simulink model "gm_mult_1"  (R2023a)
settings: Solver=FixedStepDiscrete  StartTime=0.0  StopTime=10.0  RelTol=1e-3
undefined symbols (not defined in the file or in its folder): dt
libraries: simulink x1
settings Model: Creator=szymadej  LastModifiedBy=szymadej
settings OptimizationCC: BlockReduction=off  ConditionallyExecuteInputs=off  DefaultParameterBehavior=Inlined  InheritOutputTypeSmallerThanSingle=on
settings DebuggingCC: AlgebraicLoopMsg=error  InheritedTsInSrcMsg=none  SingleTaskRateTransMsg=error  UnconnectedInputMsg=warning  UnconnectedOutputMsg=warning  UnconnectedLineMsg=warning
settings HardwareCC: ProdBitPerPointer=32  ProdBitPerSizeT=32  ProdBitPerPtrDiffT=32  ProdLargestAtomicFloat=None  ProdIntDivRoundTo=Undefined  ProdEndianess=Unspecified  ProdWordSize=32  ProdHWDeviceType=ASIC/FPGA->ASIC/FPGA  TargetBitPerLong=64  TargetBitPerPointer=64  TargetBitPerSizeT=64  TargetBitPerPtrDiffT=64  TargetLongLongMode=on  TargetIntDivRoundTo=Zero  TargetEndianess=LittleEndian  TargetWordSize=64  TargetHWDeviceType=Custom Processor->MATLAB Host Computer  ProdEqTarget=off

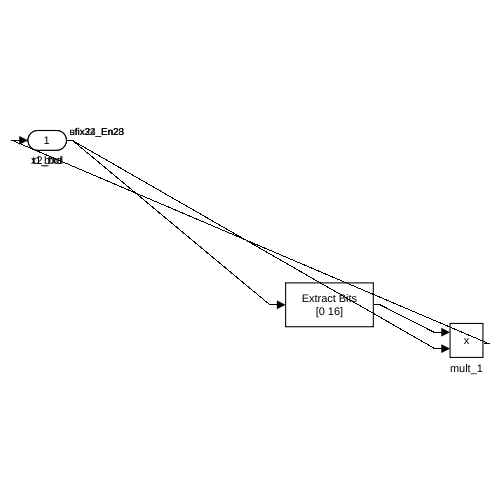
[thumbnail: Simulink's stored preview of the top-level diagram]
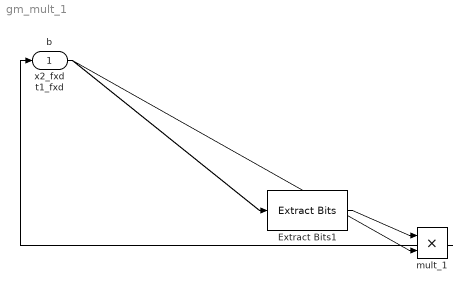
== system gm_mult_1 ==
  x2_fxd : Inport  OutDataTypeStr=fixdt(0, 24, 23)  PortDimensions=1  SampleTime=0.2
  b : Inport  Port=2  OutDataTypeStr=fixdt(1, 32, 28)  PortDimensions=1  SampleTime=0.2
  Extract Bits1 : simulink/Logic and Bit Operations/Extract Bits  bitsToExtract=Range of bits  numBits=17  bitIdxRange=[0 dt.x2_fxd.w-1]  outScalingMode=Preserve fixed-point scaling
  mult_1 : Product  OutDataTypeStr=fixdt(dt.t1_fxd.s,dt.t1_fxd.w,dt.t1_fxd.f)
  t1_fxd : Outport  SampleTime=0.2
  wires:
  x2_fxd/1 -> Extract Bits1/1
  b/1 -> mult_1/2
  Extract Bits1/1 -> mult_1/1
  mult_1/1 -> t1_fxd/1
